simulink model "S_GRAF_ELECTRO_2025_MTET_NoInt_EnvDatos_V1"  (R2017a)
settings: Solver=VariableStepAuto  StartTime=0.0  StopTime=inf  RelTol=1e-3
undefined symbols (not defined in the file or in its folder): serial
libraries: instrumentlib x2
settings Model: Creator=dricl  LastModifiedBy=dricl

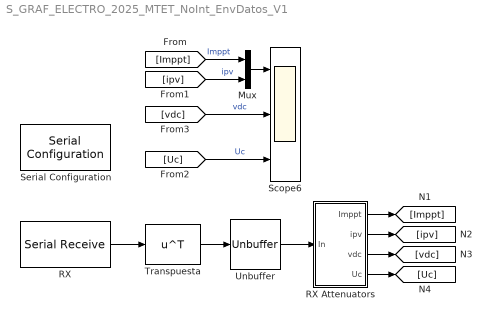
== system S_GRAF_ELECTRO_2025_MTET_NoInt_EnvDatos_V1 ==
  Mux : Mux  Inputs=2
  RX : instrumentlib/Serial Receive  ComPortMenu=COM7  ComPort=COM7  ObjConstructor=serial('COM7');  Header=SS  Terminator=EE  DataSize="[4  600]"  DataType=uint16  EnableBlockingMode=on  ActionDataUnavailable=Output custom value  CustomValue=3  SampleTime=0.03
  RX Attenuators : Subsystem
  Scope6 : Scope  NumInputPorts=3
  Serial Configuration : instrumentlib/Serial Configuration  Priority=-200000  ComPortMenu=COM7  ComPort=COM7  ObjConstructor=serial('COM7');  BaudRate=921600  DataBits=8  Parity=none  StopBits=1  FlowControl=none  Timeout=60  ByteOrder=LittleEndian
  Transpuesta : Math  Operator=transpose  SaturateOnIntegerOverflow=on
  Unbuffer : Unbuffer
  wires:
  RX/1 -> Transpuesta/1
  Transpuesta/1 -> Unbuffer/1
  Unbuffer/1 -> RX Attenuators/1(In)
  RX Attenuators/1(Imppt) -> [Imppt]
  RX Attenuators/2(ipv) -> [ipv]
  RX Attenuators/3(vdc) -> [vdc]
  [vdc] -> Scope6/2  "vdc"
  Mux/1 -> Scope6/1
  [ipv] -> Mux/2  "ipv"
  [Imppt] -> Mux/1  "Imppt"
  RX Attenuators/4(Uc) -> [Uc]
  [Uc] -> Scope6/3  "Uc"

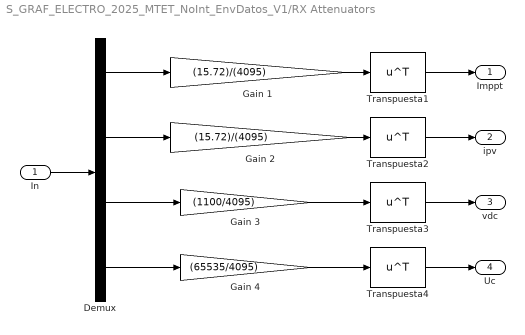
== system S_GRAF_ELECTRO_2025_MTET_NoInt_EnvDatos_V1/RX Attenuators ==
  In : Inport
  Demux : Demux
  Gain 1 : Gain  Gain=(15.72)/(4095)  OutDataTypeStr=double
  Gain 2 : Gain  Gain=(15.72)/(4095)  OutDataTypeStr=double
  Gain 3 : Gain  Gain=(1100/4095)  OutDataTypeStr=double
  Gain 4 : Gain  Gain=(65535/4095)  OutDataTypeStr=double
  Transpuesta{1..4} (4 alike) : Math  Operator=transpose  SaturateOnIntegerOverflow=on
  Imppt : Outport
  ipv : Outport  Port=2
  vdc : Outport  Port=3
  Uc : Outport  Port=4
  wires:
  Transpuesta2/1 -> ipv/1
  Gain 1/1 -> Transpuesta1/1
  Demux/1 -> Gain 1/1
  In/1 -> Demux/1
  Transpuesta1/1 -> Imppt/1
  Gain 2/1 -> Transpuesta2/1
  Demux/2 -> Gain 2/1
  Demux/3 -> Gain 3/1
  Gain 3/1 -> Transpuesta3/1
  Transpuesta3/1 -> vdc/1
  Transpuesta4/1 -> Uc/1
  Gain 4/1 -> Transpuesta4/1
  Demux/4 -> Gain 4/1
